simulink model "exp3_3"  (R2024b)
settings: Solver=VariableStepAuto  StartTime=0.0  StopTime=0.02  MaxStep=0.0002  MinStep=0.0001  RelTol=1e-4
libraries: fl_lib x108, nesl_utility x8
settings Model: Creator=ASUS  LastModifiedBy=86195
settings SolverCC: AlgebraicLoopSolver=TrustRegion
settings DataIOCC: ReturnWorkspaceOutputs=off
settings DebuggingCC: UnconnectedInputMsg=warning  UnconnectedOutputMsg=warning  UnconnectedLineMsg=warning  ArithmeticOperatorsInVariantConditions=warning
settings ModelReferenceCC: EnableRefExpFcnMdlSchedulingChecks=on
settings SFSimCC: CustomCodeUndefinedFunction=UseInterfaceOnly
settings RTWCC: GPUComputeCapability=3.5

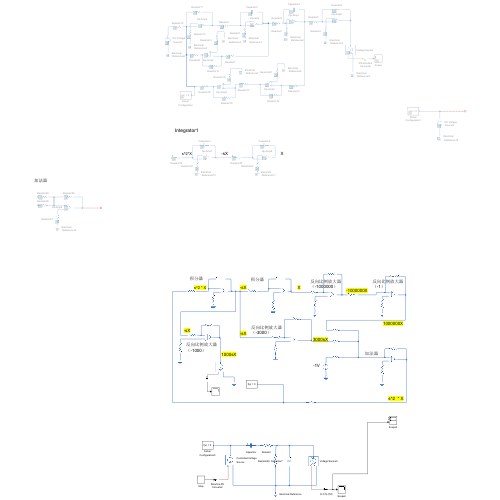
[thumbnail: Simulink's stored preview of the top-level diagram]
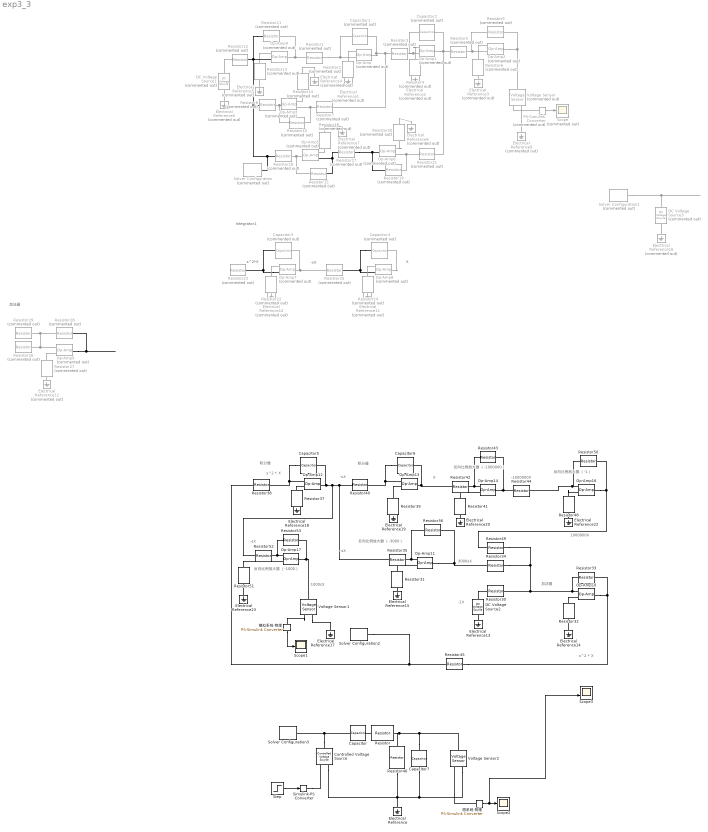
== system exp3_3 ==
  note: 反向比例放大器
      | （-3000）
  note: s^2*X
  note: Integrator1
  note: -sX
  note: X
  note: 加法器
  note: 加法器
  note: -sX
  note: s^2 * X
  note: X
  note: 3000sX
  note: 反向比例放大器
      | （-1000000）
  note: -1000000X
  note: s^2 * X
  note: 反向比例放大器
      | （-1000）
  note: 1000000X
  note: 反向比例放大器
      | （-1）
  note: -1V
  note: 积分器
  note: 积分器
  note: -sX
  note: -sX
  note: 1000sX
  Capacitor : fl_lib/Electrical/Electrical Elements/Capacitor  c=1e-6 F  r=1e-6 Ohm  g=0 1/Ohm  i_specify=off  i_priority=None  i=0 A  i_nominal_specify=off  i_nominal_value=1  i_nominal_unit=A  v_specify=off  v_priority=None  v=0 V  v_nominal_specify=off  v_nominal_value=1  v_nominal_unit=V  vc_specify=off  vc_priority=High  vc=0 V  vc_nominal_specify=off  vc_nominal_value=1  vc_nominal_unit=V
  Capacitor1 : fl_lib/Electrical/Electrical Elements/Capacitor  Commented=on  c=1000 uF  r=0 Ohm  g=0 1/Ohm  i_specify=off  i_priority=None  i=0 A  i_nominal_specify=off  i_nominal_value=1  i_nominal_unit=A  v_specify=off  v_priority=None  v=0 V  v_nominal_specify=off  v_nominal_value=1  v_nominal_unit=V  vc_specify=off  vc_priority=High  vc=0 V  vc_nominal_specify=off  vc_nominal_value=1  vc_nominal_unit=V
  Capacitor2 : fl_lib/Electrical/Electrical Elements/Capacitor  Commented=on  c=1000 uF  r=0 Ohm  g=0 1/Ohm  i_specify=off  i_priority=None  i=0 A  i_nominal_specify=off  i_nominal_value=1  i_nominal_unit=A  v_specify=off  v_priority=None  v=0 V  v_nominal_specify=off  v_nominal_value=1  v_nominal_unit=V  vc_specify=off  vc_priority=High  vc=0 V  vc_nominal_specify=off  vc_nominal_value=1  vc_nominal_unit=V
  Capacitor3 : fl_lib/Electrical/Electrical Elements/Capacitor  Commented=on  c=1 uF  r=0 Ohm  g=0 1/Ohm  i_specify=off  i_priority=None  i=0 A  i_nominal_specify=off  i_nominal_value=1  i_nominal_unit=A  v_specify=off  v_priority=None  v=0 V  v_nominal_specify=off  v_nominal_value=1  v_nominal_unit=V  vc_specify=off  vc_priority=High  vc=0 V  vc_nominal_specify=off  vc_nominal_value=1  vc_nominal_unit=V
  Capacitor4 : fl_lib/Electrical/Electrical Elements/Capacitor  Commented=on  c=1 uF  r=0 Ohm  g=0 1/Ohm  i_specify=off  i_priority=None  i=0 A  i_nominal_specify=off  i_nominal_value=1  i_nominal_unit=A  v_specify=off  v_priority=None  v=0 V  v_nominal_specify=off  v_nominal_value=1  v_nominal_unit=V  vc_specify=off  vc_priority=High  vc=0 V  vc_nominal_specify=off  vc_nominal_value=1  vc_nominal_unit=V
  Capacitor5 : fl_lib/Electrical/Electrical Elements/Capacitor  c=1 uF  r=0 Ohm  g=0 1/Ohm  i_specify=off  i_priority=None  i=0 A  i_nominal_specify=off  i_nominal_value=1  i_nominal_unit=A  v_specify=off  v_priority=None  v=0 V  v_nominal_specify=off  v_nominal_value=1  v_nominal_unit=V  vc_specify=off  vc_priority=High  vc=0 V  vc_nominal_specify=off  vc_nominal_value=1  vc_nominal_unit=V
  Capacitor6 : fl_lib/Electrical/Electrical Elements/Capacitor  c=1 uF  r=0 Ohm  g=0 1/Ohm  i_specify=off  i_priority=None  i=0 A  i_nominal_specify=off  i_nominal_value=1  i_nominal_unit=A  v_specify=off  v_priority=None  v=0 V  v_nominal_specify=off  v_nominal_value=1  v_nominal_unit=V  vc_specify=off  vc_priority=High  vc=0 V  vc_nominal_specify=off  vc_nominal_value=1  vc_nominal_unit=V
  Capacitor7 : fl_lib/Electrical/Electrical Elements/Capacitor  c=1e-6 F  r=1e-6 Ohm  g=0 1/Ohm  i_specify=off  i_priority=None  i=0 A  i_nominal_specify=off  i_nominal_value=1  i_nominal_unit=A  v_specify=off  v_priority=None  v=0 V  v_nominal_specify=off  v_nominal_value=1  v_nominal_unit=V  vc_specify=off  vc_priority=High  vc=0 V  vc_nominal_specify=off  vc_nominal_value=1  vc_nominal_unit=V
  Controlled Voltage Source : fl_lib/Electrical/Electrical Sources/Controlled Voltage Source
  DC Voltage Source1 : fl_lib/Electrical/Electrical Sources/DC Voltage Source  Commented=on  v0=1 V
  DC Voltage Source2 : fl_lib/Electrical/Electrical Sources/DC Voltage Source  v0=-1 V
  DC Voltage Source3 : fl_lib/Electrical/Electrical Sources/DC Voltage Source  Commented=on  v0=1 V
  Electrical Reference{1..12,16} (13 alike) : fl_lib/Electrical/Electrical Elements/Electrical Reference  Commented=on
  Electrical Reference{,13..15,17..20,22..23} (10 alike) : fl_lib/Electrical/Electrical Elements/Electrical Reference
  Op-Amp{,1..9} (10 alike) : fl_lib/Electrical/Electrical Elements/Op-Amp  Commented=on  outI_specify=off  outI_priority=None  outI=0 A  outI_nominal_specify=off  outI_nominal_value=1  outI_nominal_unit=A
  Op-Amp{10..14,16..17} (7 alike) : fl_lib/Electrical/Electrical Elements/Op-Amp  outI_specify=off  outI_priority=None  outI=0 A  outI_nominal_specify=off  outI_nominal_value=1  outI_nominal_unit=A
  PS-Simulink Converter : nesl_utility/PS-Simulink Converter  Commented=on  PhysicalDomain=network_engine_domain  SubClassName=ps_output  LeftPortType=input  RightPortType=output  PseudoPeriodic=off  Frequencies=[]  VectorFormat=1-D array  Unit=1  AffineConversion=off
  Resistor : fl_lib/Electrical/Electrical Elements/Resistor  R=1e3 Ohm  i_specify=off  i_priority=None  i=0 A  i_nominal_specify=off  i_nominal_value=1  i_nominal_unit=A  v_specify=off  v_priority=None  v=0 V  v_nominal_specify=off  v_nominal_value=1  v_nominal_unit=V
  Resistor{1..4,6,8,10..18,20,22,24,27} (19 alike) : fl_lib/Electrical/Electrical Elements/Resistor  Commented=on  R=1000 Ohm  i_specify=off  i_priority=None  i=0 A  i_nominal_specify=off  i_nominal_value=1  i_nominal_unit=A  v_specify=off  v_priority=None  v=0 V  v_nominal_specify=off  v_nominal_value=1  v_nominal_unit=V
  Resistor19 : fl_lib/Electrical/Electrical Elements/Resistor  Commented=on  R=10^6 Ohm  i_specify=off  i_priority=None  i=0 A  i_nominal_specify=off  i_nominal_value=1  i_nominal_unit=A  v_specify=off  v_priority=None  v=0 V  v_nominal_specify=off  v_nominal_value=1  v_nominal_unit=V
  Resistor{5,7,21,26,29} (5 alike) : fl_lib/Electrical/Electrical Elements/Resistor  Commented=on  R=1 Ohm  i_specify=off  i_priority=None  i=0 A  i_nominal_specify=off  i_nominal_value=1  i_nominal_unit=A  v_specify=off  v_priority=None  v=0 V  v_nominal_specify=off  v_nominal_value=1  v_nominal_unit=V
  Resistor23 : fl_lib/Electrical/Electrical Elements/Resistor  Commented=on  R=1e6 Ohm  i_specify=off  i_priority=None  i=0 A  i_nominal_specify=off  i_nominal_value=1  i_nominal_unit=A  v_specify=off  v_priority=None  v=0 V  v_nominal_specify=off  v_nominal_value=1  v_nominal_unit=V
  Resistor25 : fl_lib/Electrical/Electrical Elements/Resistor  Commented=on  R=1e6 Ohm  i_specify=off  i_priority=None  i=0 A  i_nominal_specify=off  i_nominal_value=1  i_nominal_unit=A  v_specify=off  v_priority=None  v=0 V  v_nominal_specify=off  v_nominal_value=1  v_nominal_unit=V
  Resistor28 : fl_lib/Electrical/Electrical Elements/Resistor  Commented=on  R=10^6 Ohm  i_specify=off  i_priority=None  i=0 A  i_nominal_specify=off  i_nominal_value=1  i_nominal_unit=A  v_specify=off  v_priority=None  v=0 V  v_nominal_specify=off  v_nominal_value=1  v_nominal_unit=V
  Resistor{30,33..35,44,49..50,52} (8 alike) : fl_lib/Electrical/Electrical Elements/Resistor  R=1e4 Ohm  i_specify=off  i_priority=None  i=0 A  i_nominal_specify=off  i_nominal_value=1  i_nominal_unit=A  v_specify=off  v_priority=None  v=0 V  v_nominal_specify=off  v_nominal_value=1  v_nominal_unit=V
  Resistor{31..32,37,39,41,45,48,51} (8 alike) : fl_lib/Electrical/Electrical Elements/Resistor  R=1000 Ohm  i_specify=off  i_priority=None  i=0 A  i_nominal_specify=off  i_nominal_value=1  i_nominal_unit=A  v_specify=off  v_priority=None  v=0 V  v_nominal_specify=off  v_nominal_value=1  v_nominal_unit=V
  Resistor36 : fl_lib/Electrical/Electrical Elements/Resistor  R=3e7 Ohm  i_specify=off  i_priority=None  i=0 A  i_nominal_specify=off  i_nominal_value=1  i_nominal_unit=A  v_specify=off  v_priority=None  v=0 V  v_nominal_specify=off  v_nominal_value=1  v_nominal_unit=V
  Resistor38 : fl_lib/Electrical/Electrical Elements/Resistor  R=1e6 Ohm  i_specify=off  i_priority=None  i=0 A  i_nominal_specify=off  i_nominal_value=1  i_nominal_unit=A  v_specify=off  v_priority=None  v=0 V  v_nominal_specify=off  v_nominal_value=1  v_nominal_unit=V
  Resistor40 : fl_lib/Electrical/Electrical Elements/Resistor  R=1e6 Ohm  i_specify=off  i_priority=None  i=0 A  i_nominal_specify=off  i_nominal_value=1  i_nominal_unit=A  v_specify=off  v_priority=None  v=0 V  v_nominal_specify=off  v_nominal_value=1  v_nominal_unit=V
  Resistor42 : fl_lib/Electrical/Electrical Elements/Resistor  R=1e3 Ohm  i_specify=off  i_priority=None  i=0 A  i_nominal_specify=off  i_nominal_value=1  i_nominal_unit=A  v_specify=off  v_priority=None  v=0 V  v_nominal_specify=off  v_nominal_value=1  v_nominal_unit=V
  Resistor43 : fl_lib/Electrical/Electrical Elements/Resistor  R=1e9 Ohm  i_specify=off  i_priority=None  i=0 A  i_nominal_specify=off  i_nominal_value=1  i_nominal_unit=A  v_specify=off  v_priority=None  v=0 V  v_nominal_specify=off  v_nominal_value=1  v_nominal_unit=V
  Resistor46 : fl_lib/Electrical/Electrical Elements/Resistor  R=1e3 Ohm  i_specify=off  i_priority=None  i=0 A  i_nominal_specify=off  i_nominal_value=1  i_nominal_unit=A  v_specify=off  v_priority=None  v=0 V  v_nominal_specify=off  v_nominal_value=1  v_nominal_unit=V
  Resistor53 : fl_lib/Electrical/Electrical Elements/Resistor  R=1e7 Ohm  i_specify=off  i_priority=None  i=0 A  i_nominal_specify=off  i_nominal_value=1  i_nominal_unit=A  v_specify=off  v_priority=None  v=0 V  v_nominal_specify=off  v_nominal_value=1  v_nominal_unit=V
  Resistor9 : fl_lib/Electrical/Electrical Elements/Resistor  Commented=on  R=10^6 Ohm  i_specify=off  i_priority=None  i=0 A  i_nominal_specify=off  i_nominal_value=1  i_nominal_unit=A  v_specify=off  v_priority=None  v=0 V  v_nominal_specify=off  v_nominal_value=1  v_nominal_unit=V
  Scope : Scope  Commented=on
  Scope1 : Scope
  Scope2 : Scope
  Scope3 : Scope  NumInputPorts=2
  Simulink-PS Converter : nesl_utility/Simulink-PS Converter  PhysicalDomain=network_engine_domain  SubClassName=ps_input  LeftPortType=input  RightPortType=output  PseudoPeriodic=off  Frequencies=[]  NoiseDistribution=none  NoiseParameters=[]  Unit=1  AffineConversion=off  FilteringAndDerivatives=provide  SimscapeFilterOrder=1  InputFilterTimeConstant=0.001  UdotUserProvided=0
  Solver Configuration : nesl_utility/Solver Configuration  Commented=on  PhysicalDomain=network_engine_domain  SubClassName=solver  LeftPortType=input  RightPortType=generic  Tones=[]  Harmonics=[]  SimulateNoise=off  Profile=off  UseLocalSampling=off  EnableSwitchedLinearOptims=on  FrequencyDomain=off  UseCCode=off  RelTol=0.001  AbsTol=1e-06  MinStep=1e-09  ToWorkspace=off  RevertToSquareIcSolve=off  NumHomotopyIterations=100  PhasorMode=off  PhasorModeNumHarmonics=1  ConsistencySolver=NEWTON_FTOL  IndexReductionMethod=DerivativeReplacement  DoDC=off  ResidualTolerance=1e-09  ConsistencyTolSource=GLOBAL  ConsistencyAbsTol=0.001  ConsistencyRelTol=0.001  ConsistencyTolFactor=0.001  UseLocalSolver=off  LocalSolverChoice=NE_BACKWARD_EULER_ADVANCER  ResolveIndetEquations=on  FunctionEvalNumThread=1  LocalSolverSampleTime=0.001  DoFixedCost=off  MaxNonlinIter=3  MaxModeIter=2  ComputeImpulses=off  ImpulseIterations=2  LinearAlgebra=auto  LinearAlgebraNumThread=0  EquationFormulation=NE_TIME_EF  DelaysMemoryBudget=1024  AutomaticFiltering=on  FilteringTimeConstant=0.001  PartitionStorageMethod=AS_NEEDED  PartitionMemoryBudget=1024  PartitionMethod=FAST  MultibodyUseLocalSolver=off  MultibodyLocalSolverChoice=ODE1  MultibodyLocalSolverSampleTime=0.001
  Solver Configuration1 : nesl_utility/Solver Configuration  Commented=on  PhysicalDomain=network_engine_domain  SubClassName=solver  LeftPortType=input  RightPortType=generic  Tones=[]  Harmonics=[]  SimulateNoise=off  Profile=off  UseLocalSampling=off  EnableSwitchedLinearOptims=on  FrequencyDomain=off  UseCCode=off  RelTol=0.001  AbsTol=0.001  MinStep=1e-09  ToWorkspace=off  RevertToSquareIcSolve=off  NumHomotopyIterations=100  PhasorMode=off  PhasorModeNumHarmonics=1  ConsistencySolver=NEWTON_XTOL_AFTER_FTOL  IndexReductionMethod=DerivativeReplacement  DoDC=off  ResidualTolerance=1e-09  ConsistencyTolSource=GLOBAL  ConsistencyAbsTol=0.001  ConsistencyRelTol=0.001  ConsistencyTolFactor=0.001  UseLocalSolver=off  LocalSolverChoice=NE_BACKWARD_EULER_ADVANCER  ResolveIndetEquations=on  FunctionEvalNumThread=1  LocalSolverSampleTime=0.001  DoFixedCost=off  MaxNonlinIter=3  MaxModeIter=2  ComputeImpulses=off  ImpulseIterations=2  LinearAlgebra=auto  LinearAlgebraNumThread=0  EquationFormulation=NE_TIME_EF  DelaysMemoryBudget=1024  AutomaticFiltering=on  FilteringTimeConstant=0.001  PartitionStorageMethod=AS_NEEDED  PartitionMemoryBudget=1024  PartitionMethod=ROBUST  MultibodyUseLocalSolver=off  MultibodyLocalSolverChoice=ODE1  MultibodyLocalSolverSampleTime=0.001
  Solver Configuration2 : nesl_utility/Solver Configuration  PhysicalDomain=network_engine_domain  SubClassName=solver  LeftPortType=input  RightPortType=generic  Tones=[]  Harmonics=[]  SimulateNoise=off  Profile=off  UseLocalSampling=off  EnableSwitchedLinearOptims=on  FrequencyDomain=off  UseCCode=off  RelTol=0.001  AbsTol=0.001  MinStep=1e-09  ToWorkspace=off  RevertToSquareIcSolve=off  NumHomotopyIterations=100  PhasorMode=off  PhasorModeNumHarmonics=1  ConsistencySolver=NEWTON_XTOL_AFTER_FTOL  IndexReductionMethod=DerivativeReplacement  DoDC=off  ResidualTolerance=1e-09  ConsistencyTolSource=GLOBAL  ConsistencyAbsTol=0.001  ConsistencyRelTol=0.001  ConsistencyTolFactor=0.001  UseLocalSolver=off  LocalSolverChoice=NE_BACKWARD_EULER_ADVANCER  ResolveIndetEquations=on  FunctionEvalNumThread=1  LocalSolverSampleTime=0.001  DoFixedCost=off  MaxNonlinIter=3  MaxModeIter=2  ComputeImpulses=off  ImpulseIterations=2  LinearAlgebra=auto  LinearAlgebraNumThread=0  EquationFormulation=NE_TIME_EF  DelaysMemoryBudget=1024  AutomaticFiltering=on  FilteringTimeConstant=0.001  PartitionStorageMethod=AS_NEEDED  PartitionMemoryBudget=1024  PartitionMethod=ROBUST  MultibodyUseLocalSolver=off  MultibodyLocalSolverChoice=ODE1  MultibodyLocalSolverSampleTime=0.001
  Solver Configuration3 : nesl_utility/Solver Configuration  PhysicalDomain=network_engine_domain  SubClassName=solver  LeftPortType=input  RightPortType=generic  Tones=[]  Harmonics=[]  SimulateNoise=off  Profile=off  UseLocalSampling=off  EnableSwitchedLinearOptims=on  FrequencyDomain=off  UseCCode=off  RelTol=0.001  AbsTol=0.001  MinStep=1e-09  ToWorkspace=off  RevertToSquareIcSolve=off  NumHomotopyIterations=100  PhasorMode=off  PhasorModeNumHarmonics=1  ConsistencySolver=NEWTON_XTOL_AFTER_FTOL  IndexReductionMethod=DerivativeReplacement  DoDC=off  ResidualTolerance=1e-09  ConsistencyTolSource=GLOBAL  ConsistencyAbsTol=0.001  ConsistencyRelTol=0.001  ConsistencyTolFactor=0.001  UseLocalSolver=off  LocalSolverChoice=NE_BACKWARD_EULER_ADVANCER  ResolveIndetEquations=on  FunctionEvalNumThread=1  LocalSolverSampleTime=0.001  DoFixedCost=off  MaxNonlinIter=3  MaxModeIter=2  ComputeImpulses=off  ImpulseIterations=2  LinearAlgebra=auto  LinearAlgebraNumThread=0  EquationFormulation=NE_TIME_EF  DelaysMemoryBudget=1024  AutomaticFiltering=on  FilteringTimeConstant=0.001  PartitionStorageMethod=AS_NEEDED  PartitionMemoryBudget=1024  PartitionMethod=ROBUST  MultibodyUseLocalSolver=off  MultibodyLocalSolverChoice=ODE1  MultibodyLocalSolverSampleTime=0.001
  Step : Step  Time=0  SampleTime=0
  Voltage Sensor : fl_lib/Electrical/Electrical Sensors/Voltage Sensor  Commented=on
  Voltage Sensor1 : fl_lib/Electrical/Electrical Sensors/Voltage Sensor
  Voltage Sensor2 : fl_lib/Electrical/Electrical Sensors/Voltage Sensor
  原系统-物理 : nesl_utility/PS-Simulink Converter  PhysicalDomain=network_engine_domain  SubClassName=ps_output  LeftPortType=input  RightPortType=output  PseudoPeriodic=off  Frequencies=[]  VectorFormat=inherit  Unit=inherit  AffineConversion=off
  模拟系统-物理 : nesl_utility/PS-Simulink Converter  PhysicalDomain=network_engine_domain  SubClassName=ps_output  LeftPortType=input  RightPortType=output  PseudoPeriodic=off  Frequencies=[]  VectorFormat=1-D array  Unit=1  AffineConversion=off
  wires:
  PS-Simulink Converter/1 -> Scope/1
  模拟系统-物理/1 -> Scope1/1
  原系统-物理/1 -> Scope3/2, Scope2/1
  Step/1 -> Simulink-PS Converter/1
  connections:
  Resistor1/RConn1 -- Capacitor1/LConn1 -- Op-Amp/LConn2
  Op-Amp/LConn1 -- Resistor2/LConn1
  Electrical Reference1/LConn1 -- Resistor2/RConn1
  Resistor3/RConn1 -- Capacitor2/LConn1 -- Op-Amp1/LConn2
  Electrical Reference2/LConn1 -- Resistor4/RConn1
  Op-Amp1/LConn1 -- Resistor4/LConn1
  Op-Amp/RConn1 -- Resistor7/LConn1 -- Resistor3/LConn1 -- Capacitor1/RConn1
  Resistor5/RConn1 -- Resistor9/LConn1 -- Op-Amp2/LConn2
  Op-Amp2/LConn1 -- Resistor6/LConn1
  Electrical Reference3/LConn1 -- Resistor6/RConn1
  Op-Amp1/RConn1 -- Capacitor2/RConn1 -- Resistor21/LConn1 -- Resistor5/LConn1
  Op-Amp2/RConn1 -- Voltage Sensor/LConn1 -- Resistor9/RConn1
  Op-Amp4/LConn1 -- Resistor13/LConn1
  Electrical Reference5/LConn1 -- Resistor13/RConn1
  Electrical Reference6/LConn1 -- DC Voltage Source1/RConn1
  DC Voltage Source1/LConn1 -- Resistor12/LConn1
  Op-Amp4/RConn1 -- Resistor11/RConn1 -- Resistor1/LConn1
  Resistor7/RConn1 -- Resistor10/LConn1 -- Op-Amp3/LConn2
  Resistor8/LConn1 -- Op-Amp3/RConn1 -- Resistor10/RConn1
  Resistor11/LConn1 -- Solver Configuration/RConn1 -- Resistor18/RConn1 -- Resistor8/RConn1 -- Resistor12/RConn1 -- Op-Amp4/LConn2
  Op-Amp3/LConn1 -- Resistor14/RConn1
  Resistor14/LConn1 -- Electrical Reference4/LConn1
  Resistor15/LConn1 -- Resistor17/RConn1 -- Op-Amp5/LConn2
  Resistor18/LConn1 -- Resistor15/RConn1 -- Op-Amp5/RConn1
  Resistor16/LConn1 -- Electrical Reference7/LConn1
  Op-Amp5/LConn1 -- Resistor16/RConn1
  Resistor21/RConn1 -- Resistor19/LConn1 -- Op-Amp6/LConn2
  Op-Amp6/RConn1 -- Resistor17/LConn1 -- Resistor19/RConn1
  Op-Amp6/LConn1 -- Resistor20/RConn1
  Resistor20/LConn1 -- Electrical Reference8/LConn1
  Voltage Sensor/RConn2 -- Electrical Reference9/LConn1
  Voltage Sensor/RConn1 -- PS-Simulink Converter/LConn1
  Op-Amp7/LConn2 -- Resistor23/RConn1 -- Capacitor3/LConn1
  Op-Amp7/RConn1 -- Capacitor3/RConn1 -- Resistor25/LConn1
  Op-Amp7/LConn1 -- Resistor22/LConn1
  Electrical Reference10/LConn1 -- Resistor22/RConn1
  Capacitor4/LConn1 -- Op-Amp8/LConn2 -- Resistor25/RConn1
  Op-Amp8/RConn1 -- Capacitor4/RConn1
  Op-Amp8/LConn1 -- Resistor24/LConn1
  Electrical Reference11/LConn1 -- Resistor24/RConn1
  Resistor28/RConn1 -- Op-Amp9/RConn1
  Resistor28/LConn1 -- Resistor29/RConn1 -- Op-Amp9/LConn2 -- Resistor26/RConn1
  Electrical Reference12/LConn1 -- Resistor27/RConn1
  Resistor27/LConn1 -- Op-Amp9/LConn1
  Electrical Reference13/LConn1 -- DC Voltage Source2/RConn1
  DC Voltage Source2/LConn1 -- Resistor30/LConn1
  Op-Amp10/RConn1 -- Resistor45/LConn1 -- Resistor33/RConn1
  Op-Amp10/LConn2 -- Resistor33/LConn1 -- Resistor34/RConn1 -- Resistor49/RConn1 -- Resistor30/RConn1
  Resistor32/LConn1 -- Op-Amp10/LConn1
  Electrical Reference14/LConn1 -- Resistor32/RConn1
  Electrical Reference15/LConn1 -- Resistor31/RConn1
  Resistor31/LConn1 -- Op-Amp11/LConn1
  Resistor35/RConn1 -- Resistor36/LConn1 -- Op-Amp11/LConn2
  Op-Amp11/RConn1 -- Resistor36/RConn1 -- Resistor34/LConn1
  DC Voltage Source3/LConn1 -- Solver Configuration1/RConn1
  Electrical Reference16/LConn1 -- DC Voltage Source3/RConn1
  Voltage Sensor1/RConn2 -- Electrical Reference17/LConn1
  Voltage Sensor1/RConn1 -- 模拟系统-物理/LConn1
  Op-Amp12/RConn1 -- Resistor52/LConn1 -- Resistor35/LConn1 -- Resistor40/LConn1 -- Capacitor5/RConn1
  Capacitor6/LConn1 -- Resistor40/RConn1 -- Op-Amp13/LConn2
  Op-Amp13/RConn1 -- Capacitor6/RConn1 -- Resistor42/LConn1
  Capacitor5/LConn1 -- Op-Amp12/LConn2 -- Resistor38/RConn1
  Op-Amp13/LConn1 -- Resistor39/LConn1
  Op-Amp12/LConn1 -- Resistor37/LConn1
  Electrical Reference18/LConn1 -- Resistor37/RConn1
  Electrical Reference19/LConn1 -- Resistor39/RConn1
  Op-Amp14/RConn1 -- Resistor44/LConn1 -- Resistor43/RConn1
  Resistor42/RConn1 -- Resistor43/LConn1 -- Op-Amp14/LConn2
  Resistor41/LConn1 -- Op-Amp14/LConn1
  Electrical Reference20/LConn1 -- Resistor41/RConn1
  Resistor38/LConn1 -- Resistor45/RConn1 -- Solver Configuration2/RConn1
  Op-Amp17/LConn2 -- Resistor52/RConn1 -- Resistor53/LConn1
  Resistor51/LConn1 -- Op-Amp17/LConn1
  Op-Amp17/RConn1 -- Voltage Sensor1/LConn1 -- Resistor53/RConn1
  Electrical Reference23/LConn1 -- Resistor51/RConn1
  Resistor48/LConn1 -- Op-Amp16/LConn1
  Electrical Reference22/LConn1 -- Resistor48/RConn1
  Op-Amp16/LConn2 -- Resistor44/RConn1 -- Resistor50/LConn1
  Op-Amp16/RConn1 -- Resistor50/RConn1 -- Resistor49/LConn1
  Controlled Voltage Source/LConn1 -- Capacitor/LConn1 -- Solver Configuration3/RConn1
  Voltage Sensor2/RConn2 -- Controlled Voltage Source/RConn2 -- Electrical Reference/LConn1 -- Resistor46/RConn1 -- Capacitor7/RConn1
  Capacitor7/LConn1 -- Resistor/RConn1 -- Resistor46/LConn1 -- Voltage Sensor2/LConn1
  原系统-物理/LConn1 -- Voltage Sensor2/RConn1
  Capacitor/RConn1 -- Resistor/LConn1
  Simulink-PS Converter/RConn1 -- Controlled Voltage Source/RConn1
